simulink model "untitled"  (Simulink 7.7)
settings: Solver=ode45  StartTime=0.0  StopTime=10.0  RelTol=1e-3
libraries: cstblocks x2
settings Model: Creator=Muhammad Ali khan  LastModifiedBy=Muhammad Ali khan

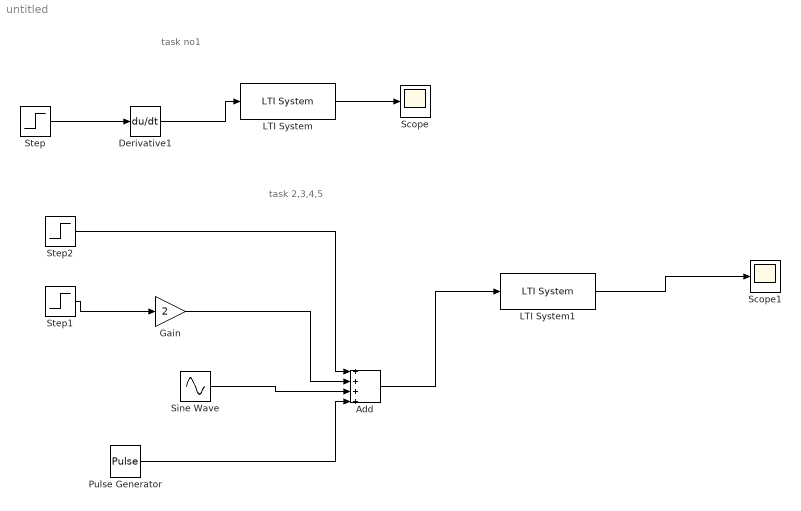
== system untitled ==
  note: task no1
  note: task 2,3,4,5
  Add : Sum  Inputs=++++
  Derivative1 : Derivative
  Gain : Gain  Gain=2
  LTI System : cstblocks/LTI System  SystemSampleTime=-1  sys="tf(100,[1  4 20])"  IC=[]
  LTI System1 : cstblocks/LTI System  SystemSampleTime=-1  sys="tf(100,[1  4 20])"  IC=[]
  Pulse Generator : DiscretePulseGenerator  PulseType=Time based  Amplitude=2  Period=10  PulseWidth=5
  Scope : Scope
  Scope1 : Scope
      settings: TimeRange=40
  Sine Wave : Sin  SampleTime=0
  Step : Step  SampleTime=0
  Step1 : Step  Time=5  SampleTime=0
  Step2 : Step  SampleTime=0
  wires:
  Step/1 -> Derivative1/1
  LTI System/1 -> Scope/1
  Step1/1 -> Gain/1
  Gain/1 -> Add/2
  Step2/1 -> Add/1
  Pulse Generator/1 -> Add/4
  Sine Wave/1 -> Add/3
  Add/1 -> LTI System1/1
  Derivative1/1 -> LTI System/1
  LTI System1/1 -> Scope1/1
